simulink model "ps11_input_design_tikh"  (R2014b)
settings: Solver=ode45  StartTime=0.0  StopTime=10*h  RelTol=1e-3
values from neighbouring files (symbols this model uses):
  A = [0, 0, 0 ... (first row only)    [Apollo_LM_design.m]    (also in Apollo_LM_design_observer.m; Apollo_LM_share.m; L11.m = [-2, -0.02, 0; 1, 0, 0; 0, 1, 0]; cart-oscillator-input-design.m = [0, 1; -w^2, 0])
  B = [k1;0;0]    [Apollo_LM_design.m]    (also in Apollo_LM_design_observer.m; Apollo_LM_share.m; L11.m = [1;0;0]; cart-oscillator-input-design.m = [0;w^2])
  h = 1    [Apollo_LM_design.m]    (also in Apollo_LM_design_observer.m; Apollo_LM_share.m = 0.25; L11.m = 0.1; cart-oscillator-input-design.m = 0.5)
libraries: simulink x2
settings Model: Creator=kjartan  LastModifiedBy=kjartan

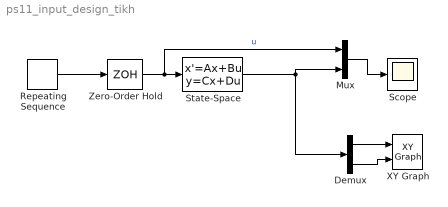
== system ps11_input_design_tikh ==
  Demux : Demux  Outputs=2
  Mux : Mux  Inputs=2
  Repeating Sequence : simulink/Sources/Repeating Sequence  rep_seq_t=t  rep_seq_y=uu
  Scope : Scope
      settings: ShowLegends=on
  State-Space : StateSpace  A=A  B=B  C=eye(2)  D=zeros(2,1)  X0=0
  XY Graph : simulink/Sinks/XY Graph  xmin=-1  xmax=1  ymin=-1  ymax=1  st=-1
  Zero-Order Hold : ZeroOrderHold  SampleTime=h
  wires:
  Demux/1 -> XY Graph/1
  Demux/2 -> XY Graph/2
  State-Space/1 -> Mux/2, Demux/1
  Zero-Order Hold/1 -> Mux/1, State-Space/1  "u"
  Repeating Sequence/1 -> Zero-Order Hold/1
  Mux/1 -> Scope/1
